simulink model "Dynamic_Simulation"  (R2016b)
settings: Solver=VariableStepAuto  StartTime=0.0  StopTime=10.0  RelTol=1e-3
settings Model: Creator=Dylan  LastModifiedBy=Dylan

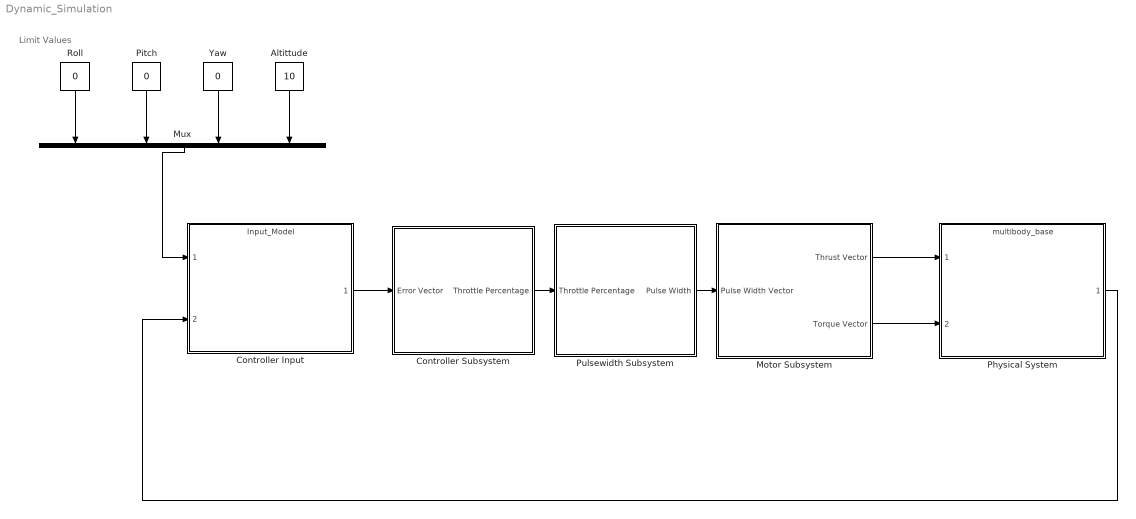
== system Dynamic_Simulation ==
  note: Limit Values
  Altittude : Constant  Value=10
  Controller Input : ModelReference  ModelNameDialog=Input_Model.slx  SimulationMode=Normal  ModelReferenceVersion=1.12
  Controller Subsystem : Subsystem
  Motor Subsystem : Subsystem
  Mux : Mux
  Physical System : ModelReference  ModelNameDialog=multibody_base.slx  SimulationMode=Normal  Variant=on  ModelReferenceVersion=1.17
      settings: AttributesFormatString=%<ActiveVariant>
  Pitch : Constant  Value=0
  Pulsewidth Subsystem : Subsystem
  Roll : Constant  Value=0
  Yaw : Constant  Value=0
  wires:
  Motor Subsystem/2(Torque Vector) -> Physical System/2
  Motor Subsystem/1(Thrust Vector) -> Physical System/1
  Physical System/1 -> Controller Input/2
  Controller Input/1 -> Controller Subsystem/1(Error Vector)
  Mux/1 -> Controller Input/1
  Altittude/1 -> Mux/4
  Yaw/1 -> Mux/3
  Pitch/1 -> Mux/2
  Roll/1 -> Mux/1
  Pulsewidth Subsystem/1(Pulse Width) -> Motor Subsystem/1(Pulse Width Vector)
  Controller Subsystem/1(Throttle Percentage) -> Pulsewidth Subsystem/1(Throttle Percentage)

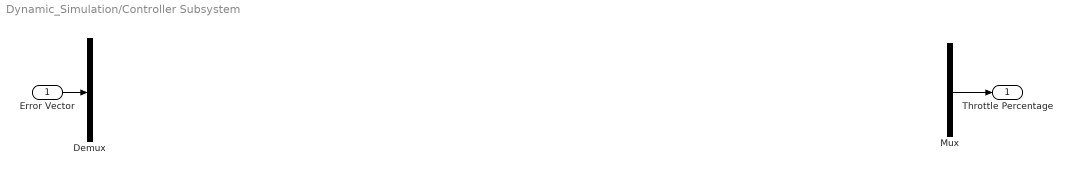
== system Dynamic_Simulation/Controller Subsystem ==
  Error Vector : Inport
  Demux : Demux
  Mux : Mux
  Throttle Percentage : Outport
  wires:
  Error Vector/1 -> Demux/1
  Mux/1 -> Throttle Percentage/1

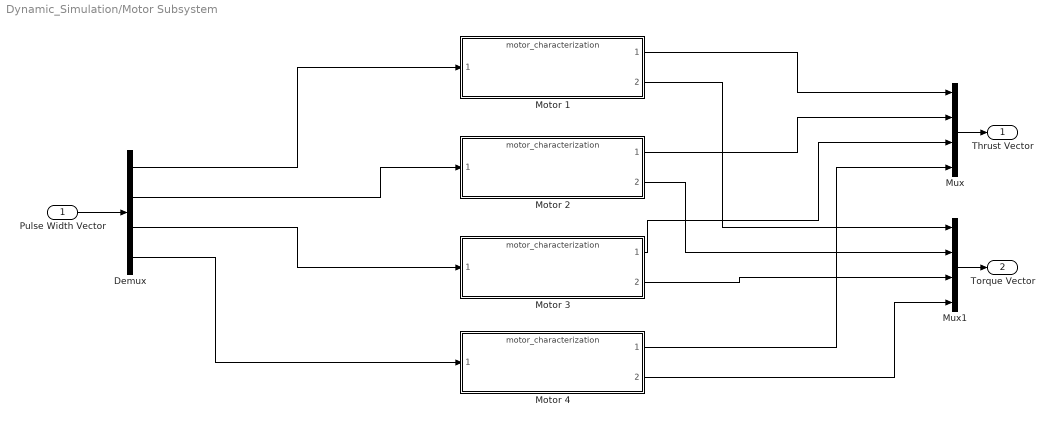
== system Dynamic_Simulation/Motor Subsystem ==
  Pulse Width Vector : Inport
  Demux : Demux
  Motor {1..4} (4 alike) : ModelReference  ModelNameDialog=motor_characterization.slx  SimulationMode=Normal  Variant=on  ModelReferenceVersion=1.7
      settings: AttributesFormatString=%<ActiveVariant>
  Mux : Mux
  Mux1 : Mux
  Thrust Vector : Outport
  Torque Vector : Outport  Port=2
  wires:
  Pulse Width Vector/1 -> Demux/1
  Mux/1 -> Thrust Vector/1
  Mux1/1 -> Torque Vector/1
  Demux/1 -> Motor 1/1
  Demux/2 -> Motor 2/1
  Demux/3 -> Motor 3/1
  Demux/4 -> Motor 4/1
  Motor 1/1 -> Mux/1
  Motor 2/1 -> Mux/2
  Motor 3/1 -> Mux/3
  Motor 4/1 -> Mux/4
  Motor 1/2 -> Mux1/1
  Motor 2/2 -> Mux1/2
  Motor 3/2 -> Mux1/3
  Motor 4/2 -> Mux1/4

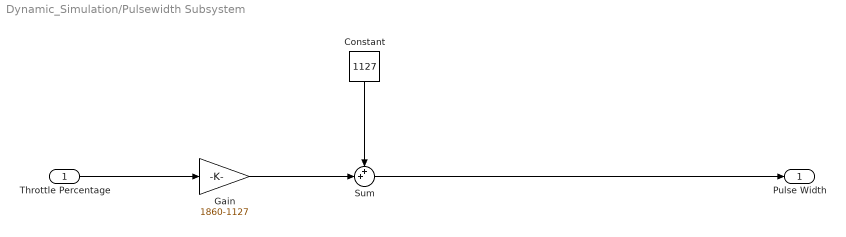
== system Dynamic_Simulation/Pulsewidth Subsystem ==
  Throttle Percentage : Inport
  Constant : Constant  Value=1127
  Gain : Gain  Gain=1860-1127
  Sum : Sum  Inputs=++|
  Pulse Width : Outport
  wires:
  Throttle Percentage/1 -> Gain/1
  Constant/1 -> Sum/1
  Gain/1 -> Sum/2
  Sum/1 -> Pulse Width/1
